simulink library "csu_elk_est_landed_kinematics_mtv_lib"  (R2014b)
settings: Solver=ode45  StartTime=0.0  StopTime=10.0  RelTol=1e-3
undefined symbols (not defined in the file or in its folder): elk_body_base_to_origin, elk_launchstand_height, integrating, kfl_target_site_planet_fixed, landed
libraries: simulink x10, util_common_lib x6, util_event_lib x4, util_info_lib x1
settings Model: Creator=escrane  LastModifiedBy=mstewart

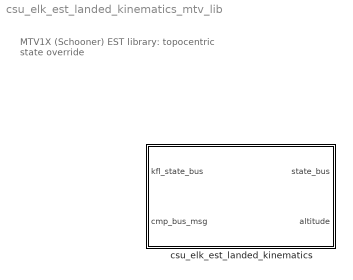
== system csu_elk_est_landed_kinematics_mtv_lib ==
  note: MTV1X (Schooner) EST library:
      | topocentric state override
  csu_elk_est_landed_kinematics : Subsystem

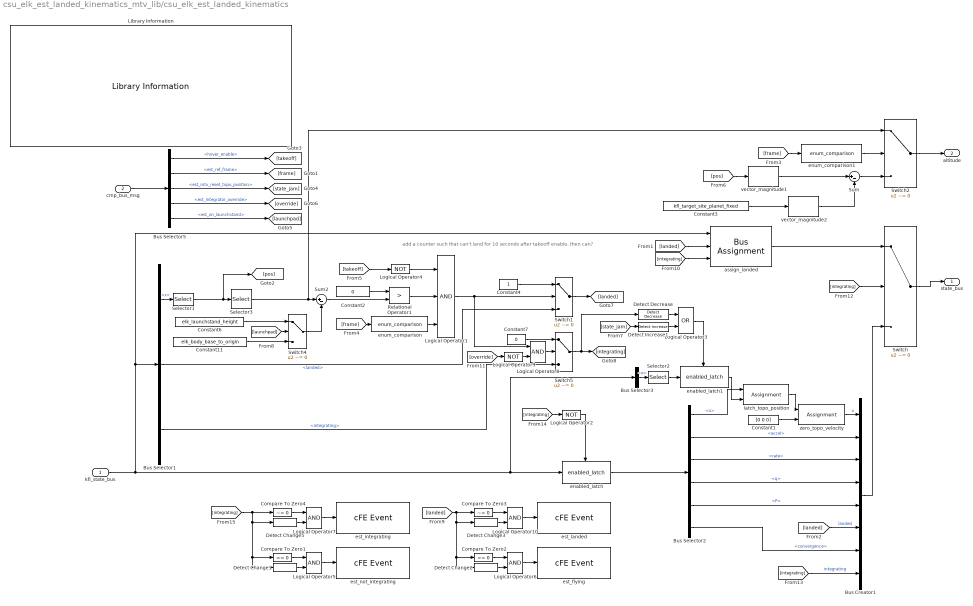
== system csu_elk_est_landed_kinematics_mtv_lib/csu_elk_est_landed_kinematics ==
  note: add a counter such that can't land for 10 seconds after takeoff enable, then can?
  kfl_state_bus : Inport
  cmp_bus_msg : Inport  Port=2
  Bus Creator1 : BusCreator  Inputs=8
  Bus Selector1 : BusSelector  OutputSignals=x,landed,integrating
  Bus Selector2 : BusSelector  OutputSignals=x,accel,rate,q,P,convergence
  Bus Selector3 : BusSelector  OutputSignals=x
  Bus Selector5 : BusSelector  OutputSignals=hover_enable,est_ref_frame,est_mtv_reset_topo_position,est_integrator_override,est_on_launchstand
  Compare To Zero1 : simulink/Logic and Bit Operations/Compare To Zero  relop===  OutDataTypeStr=boolean
  Compare To Zero2 : simulink/Logic and Bit Operations/Compare To Zero  relop===  OutDataTypeStr=boolean
  Compare To Zero3 : simulink/Logic and Bit Operations/Compare To Zero  relop=~=  OutDataTypeStr=boolean
  Compare To Zero4 : simulink/Logic and Bit Operations/Compare To Zero  relop=~=  OutDataTypeStr=boolean
  Constant1 : Constant  Value=[0 0 0]
  Constant11 : Constant  Value=elk_body_base_to_origin  VectorParams1D=off
  Constant2 : Constant  Value=0
  Constant3 : Constant  Value=kfl_target_site_planet_fixed  VectorParams1D=off
  Constant4 : Constant
  Constant6 : Constant  Value=elk_launchstand_height  VectorParams1D=off
  Constant7 : Constant  Value=0
  Detect Change{1..3,5} (4 alike) : simulink/Logic and Bit Operations/Detect Change  vinit=0  InputProcessing=Inherited  OutDataTypeStr=boolean
  Detect Decrease : simulink/Logic and Bit Operations/Detect Decrease  vinit=1  InputProcessing=Inherited  OutDataTypeStr=boolean
  Detect Increase1 : simulink/Logic and Bit Operations/Detect Increase  vinit=0  InputProcessing=Inherited  OutDataTypeStr=boolean
  Library Information : util_info_lib/Library Information  owner='escrane'
  Logical Operator{5..8,10} (5 alike) : Logic  AllPortsSameDT=off  OutDataTypeStr=boolean
  Logical Operator1 : Logic  Inputs=3  AllPortsSameDT=off  OutDataTypeStr=boolean
  Logical Operator2 : Logic  Operator=NOT  AllPortsSameDT=off  OutDataTypeStr=boolean
  Logical Operator3 : Logic  Operator=OR  AllPortsSameDT=off  OutDataTypeStr=boolean
  Logical Operator4 : Logic  Operator=NOT  AllPortsSameDT=off  OutDataTypeStr=boolean
  Logical Operator9 : Logic  Operator=NOT  AllPortsSameDT=off  OutDataTypeStr=boolean
  Relational Operator1 : RelationalOperator  Operator=>  OutDataTypeStr=boolean
  Selector1 : Selector  InputPortWidth=kfl_n_state  Indices=kfl_pos_index
  Selector2 : Selector  InputPortWidth=kfl_n_state  Indices=kfl_pos_index
  Selector3 : Selector  InputPortWidth=3  Indices=[3]
  Sum : Sum  Inputs=|+-
  Sum2 : Sum  Inputs=|+-
  Switch{,1..2,4..5} (5 alike) : Switch  Criteria=u2 ~= 0
  assign_landed : BusAssignment  AssignedSignals=landed,integrating
  enabled_latch : util_common_lib/enabled_latch  initial_output=0
  enabled_latch1 : util_common_lib/enabled_latch  initial_output=0
  enum_comparison : util_common_lib/enum_comparison  comparison_type===
  enum_comparison1 : util_common_lib/enum_comparison  comparison_type===
  est_flying : util_event_lib/cFE Event  event_message='EST declares vehicle FLYING'  event_id=20  event_severity=INFORMATION  event_use_enums=off  event_enum_types={}
  est_integrating : util_event_lib/cFE Event  event_message='EST integrating position from MEMS'  event_id=20  event_severity=INFORMATION  event_use_enums=off  event_enum_types={}
  est_landed : util_event_lib/cFE Event  event_message='EST declares vehicle LANDED'  event_id=20  event_severity=INFORMATION  event_use_enums=off  event_enum_types={}
  est_not_integrating : util_event_lib/cFE Event  event_message='EST propagating position on surface'  event_id=20  event_severity=INFORMATION  event_use_enums=off  event_enum_types={}
  latch_topo_position : Assignment  Indices=kfl_pos_index
  vector_magnitude1 : util_common_lib/vector_magnitude  SystemSampleTime=-1
  vector_magnitude2 : util_common_lib/vector_magnitude  SystemSampleTime=-1
  zero_topo_velocity : Assignment  Indices=kfl_vel_index
  state_bus : Outport
  altitude : Outport  Port=2
  wires:
  Logical Operator4/1 -> Logical Operator1/1
  Bus Selector5/1 -> [takeoff]  "<hover_enable>"
  Detect Change2/1 -> Logical Operator6/2
  Compare To Zero2/1 -> Logical Operator6/1
  Logical Operator6/1 -> est_flying/1
  [landed] -> Compare To Zero3/1, Detect Change2/1, Compare To Zero2/1, Detect Change3/1
  Detect Change3/1 -> Logical Operator10/2
  Compare To Zero3/1 -> Logical Operator10/1
  Logical Operator10/1 -> est_landed/1
  Switch1/1 -> [landed]
  [integrating] -> Logical Operator2/1
  Logical Operator2/1 -> enabled_latch/Enable
  [integrating] -> Bus Creator1/8  "integrating"
  assign_landed/1 -> Switch/1
  [integrating] -> assign_landed/3
  Switch5/1 -> [integrating], Detect Decrease/1
  Bus Selector1/3 -> Switch5/3  "<integrating>"
  Logical Operator9/1 -> Logical Operator8/2
  [override] -> Logical Operator9/1
  Logical Operator8/1 -> Switch5/2
  Constant7/1 -> Switch5/1
  Detect Change1/1 -> Logical Operator5/2
  Compare To Zero1/1 -> Logical Operator5/1
  Logical Operator5/1 -> est_not_integrating/1
  [integrating] -> Compare To Zero4/1, Detect Change5/1, Detect Change1/1, Compare To Zero1/1
  Detect Change5/1 -> Logical Operator7/2
  Compare To Zero4/1 -> Logical Operator7/1
  Logical Operator7/1 -> est_integrating/1
  Bus Selector5/5 -> [launchpad]  "<est_on_launchstand>"
  [launchpad] -> Switch4/2
  Constant6/1 -> Switch4/1
  Constant11/1 -> Switch4/3
  Switch4/1 -> Sum2/2
  Bus Selector5/4 -> [override]  "<est_integrator_override>"
  Switch2/1 -> altitude/1
  [state_jam] -> Detect Increase1/1
  Bus Selector5/3 -> [state_jam]  "<est_mtv_reset_topo_position>"
  Detect Increase1/1 -> Logical Operator3/2
  Detect Decrease/1 -> Logical Operator3/1
  enabled_latch1/1 -> latch_topo_position/2
  Logical Operator3/1 -> enabled_latch1/Enable
  Selector2/1 -> enabled_latch1/1
  Bus Selector3/1 -> Selector2/1  "<x>"
  latch_topo_position/1 -> zero_topo_velocity/1
  Bus Selector2/6 -> Bus Creator1/7  "<convergence>"
  Constant3/1 -> vector_magnitude2/1
  vector_magnitude1/1 -> Sum/1
  [pos] -> vector_magnitude1/1
  enum_comparison1/1 -> Switch2/2
  [frame] -> enum_comparison1/1
  Selector3/1 -> Switch2/1, Sum2/1
  [takeoff] -> Logical Operator4/1
  Relational Operator1/1 -> Logical Operator1/2
  enum_comparison/1 -> Logical Operator1/3
  Bus Selector1/2 -> Switch1/3  "<landed>"
  Constant4/1 -> Switch1/1
  Logical Operator1/1 -> Switch1/2, Logical Operator8/1
  [landed] -> assign_landed/2
  [landed] -> Bus Creator1/6  "landed"
  Sum2/1 -> Relational Operator1/2
  Constant2/1 -> Relational Operator1/1
  Bus Creator1/1 -> Switch/3
  kfl_state_bus/1 -> Bus Selector1/1, assign_landed/1, Bus Selector3/1, enabled_latch/1
  [integrating] -> Switch/2
  zero_topo_velocity/1 -> Bus Creator1/1  "x"
  Constant1/1 -> zero_topo_velocity/2
  enabled_latch/1 -> Bus Selector2/1
  Bus Selector2/1 -> latch_topo_position/1  "<x>"
  Bus Selector2/5 -> Bus Creator1/5  "<P>"
  Bus Selector2/2 -> Bus Creator1/2  "<accel>"
  Switch/1 -> state_bus/1
  Bus Selector2/3 -> Bus Creator1/3  "<rate>"
  Bus Selector2/4 -> Bus Creator1/4  "<q>"
  Selector1/1 -> Selector3/1, [pos]
  Bus Selector1/1 -> Selector1/1  "<x>"
  Bus Selector5/2 -> [frame]  "<est_ref_frame>"
  cmp_bus_msg/1 -> Bus Selector5/1
  [frame] -> enum_comparison/1
  Sum/1 -> Switch2/3
  vector_magnitude2/1 -> Sum/2
